simulink subsystem "Regler"  (R2021b)
settings: Solver=VariableStepAuto  StartTime=0.0  StopTime=10.0  RelTol=1e-3
undefined symbols (not defined in the file or in its folder): RegPar
settings Model: Creator=tim  LastModifiedBy=tim

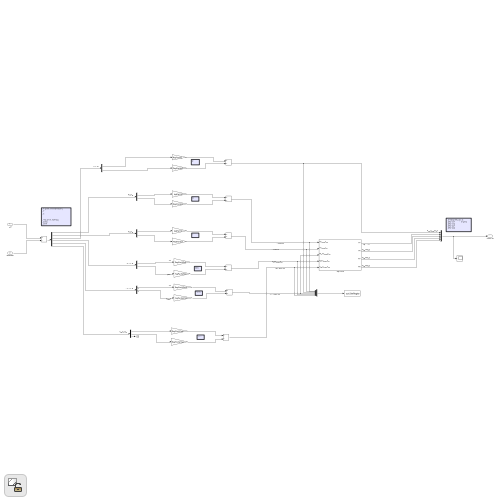
[thumbnail: Simulink's stored preview of the top-level diagram]
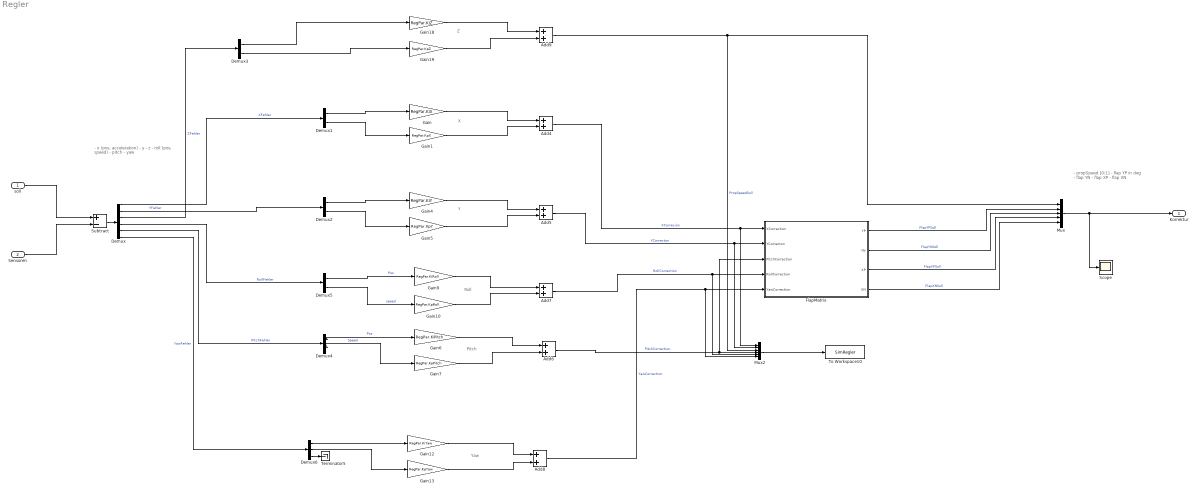
== system Regler ==
  note: Z
  note: - x (pos, acceleration)
      | - y
      | - z
      |
      |
      | - roll (pos, speed)
      | - pitch
      | - yaw
  note: Y
  note: X
  note: Pitch
  note: Roll
  note: Yaw
  note: - propSpeed [0;1]
      | - flap YP          in deg
      | - flap YN
      | - flap XP
      | - flap XN
  soll : Inport
  Sensoren : Inport  Port=2
  Add{4..9} (6 alike) : Sum
  Demux : Demux  Outputs=[2 2 2 2 2 2 ]
  Demux{1..5} (5 alike) : Demux  Outputs=2
  Demux6 : Demux  Outputs=3
  FlapMatrix : Subsystem
  Gain : Gain  Gain=RegPar.KiX
  Gain1 : Gain  Gain=RegPar.KpX
  Gain10 : Gain  Gain=RegPar.KpRoll
  Gain12 : Gain  Gain=RegPar.KiYaw
  Gain13 : Gain  Gain=RegPar.KpYaw
  Gain18 : Gain  Gain=RegPar.KiZ
  Gain19 : Gain  Gain=RegPar.KpZ
  Gain4 : Gain  Gain=RegPar.KiY
  Gain5 : Gain  Gain=RegPar.KpY
  Gain6 : Gain  Gain=RegPar.KiPitch
  Gain7 : Gain  Gain=RegPar.KpPitch
  Gain9 : Gain  Gain=RegPar.KiRoll
  Mux : Mux  Inputs=5
  Mux2 : Mux  Inputs=6
  Scope : Scope
  Subtract : Sum  Inputs=+-
  Terminator5 : Terminator
  To Workspace10 : ToWorkspace  VariableName=SimRegler  SaveFormat=Timeseries  SampleTime=-1
  Korrektur : Outport
  wires:
  soll/1 -> Subtract/1
  Mux/1 -> Korrektur/1, Scope/1
  Add9/1 -> Mux/1, Mux2/3  "PropSpeedSoll"
  Subtract/1 -> Demux/1
  Demux/1 -> Demux1/1  "XFehler"
  Demux/2 -> Demux2/1  "YFehler"
  Demux/3 -> Demux3/1  "ZFehler"
  Demux/4 -> Demux5/1  "RollFehler"
  Demux4/1 -> Gain6/1  "Pos"
  Demux4/2 -> Gain7/1  "Speed"
  Demux5/1 -> Gain9/1  "Pos"
  Demux5/2 -> Gain10/1  "speed"
  Add4/1 -> FlapMatrix/1(XCorrection), Mux2/1  "XCorrecion"
  Add5/1 -> FlapMatrix/2(YCorrecton), Mux2/2  "YCorrecton"
  Add7/1 -> Mux2/5, FlapMatrix/4(RollCorrection)  "RollCorrection"
  FlapMatrix/4(XN) -> Mux/5  "FlapXNSoll"
  FlapMatrix/3(XP) -> Mux/4  "FlapXPSoll"
  FlapMatrix/2(YN) -> Mux/3  "FlapYNSoll"
  FlapMatrix/1(YP) -> Mux/2  "FlapYPSoll"
  Sensoren/1 -> Subtract/2
  Add6/1 -> Mux2/4, FlapMatrix/3(PitchCorrection)  "PitchCorrection"
  Demux/6 -> Demux6/1  "YawFehler"
  Demux/5 -> Demux4/1  "PitchFehler"
  Gain/1 -> Add4/1
  Gain1/1 -> Add4/2
  Demux1/2 -> Gain1/1
  Demux1/1 -> Gain/1
  Gain4/1 -> Add5/1
  Demux2/1 -> Gain4/1
  Demux2/2 -> Gain5/1
  Gain5/1 -> Add5/2
  Gain6/1 -> Add6/1
  Gain7/1 -> Add6/2
  Gain9/1 -> Add7/1
  Gain10/1 -> Add7/2
  Add8/1 -> Mux2/6, FlapMatrix/5(YawCorrection)  "YawCorrection"
  Gain12/1 -> Add8/1
  Gain13/1 -> Add8/2
  Demux6/2 -> Gain13/1
  Demux6/1 -> Gain12/1
  Gain18/1 -> Add9/1
  Gain19/1 -> Add9/2
  Demux3/2 -> Gain19/1
  Demux3/1 -> Gain18/1
  Demux6/3 -> Terminator5/1
  Mux2/1 -> To Workspace10/1

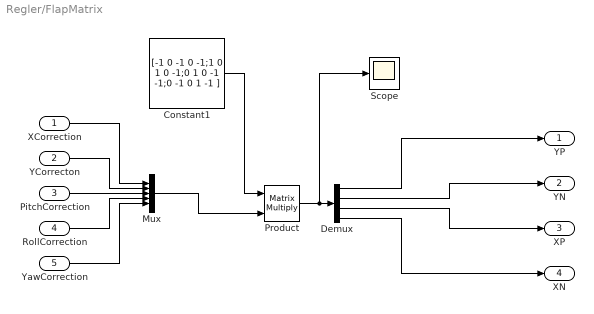
== system Regler/FlapMatrix ==
  XCorrection : Inport
  YCorrecton : Inport  Port=2
  PitchCorrection : Inport  Port=3
  RollCorrection : Inport  Port=4
  YawCorrection : Inport  Port=5
  Constant1 : Constant  Value=[-1 0 -1 0 -1;1 0 1 0 -1;0 1 0 -1 -1;0 -1 0 1 -1 ]
  Demux : Demux
  Mux : Mux  Inputs=5
  Product : Product  Multiplication=Matrix(*)
  Scope : Scope
  YP : Outport
  YN : Outport  Port=2
  XP : Outport  Port=3
  XN : Outport  Port=4
  wires:
  Demux/4 -> XN/1
  Demux/3 -> XP/1
  Demux/2 -> YN/1
  Demux/1 -> YP/1
  Product/1 -> Demux/1, Scope/1
  Constant1/1 -> Product/1
  Mux/1 -> Product/2
  YawCorrection/1 -> Mux/5
  RollCorrection/1 -> Mux/4
  PitchCorrection/1 -> Mux/3
  YCorrecton/1 -> Mux/2
  XCorrection/1 -> Mux/1
